simulink model "Decoder_3_8"  (R2018a)
settings: Solver=VariableStepAuto  StartTime=0.0  StopTime=10.0  RelTol=1e-3
settings Model: Creator=midog  LastModifiedBy=midog

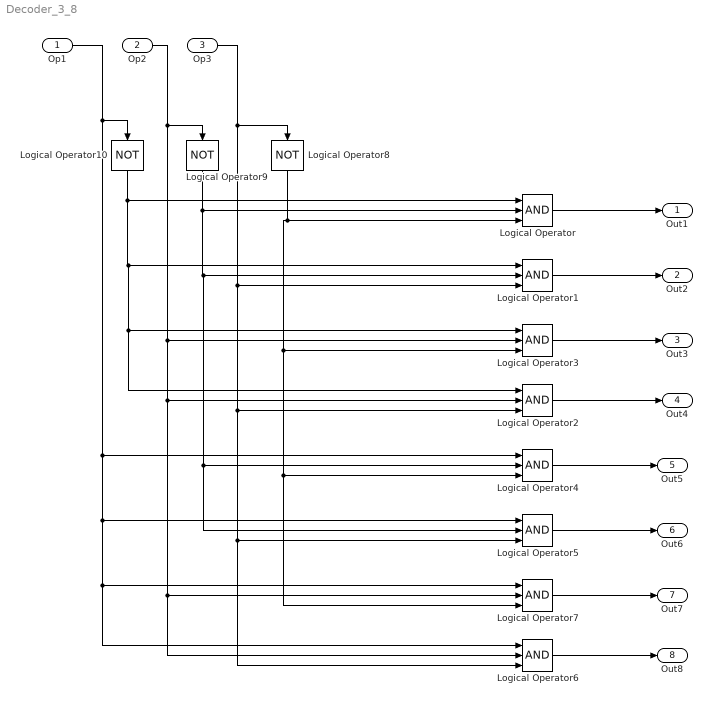
== system Decoder_3_8 ==
  Op1 : Inport  OutMin=0  OutMax=1
  Op2 : Inport  Port=2  OutMin=0  OutMax=1
  Op3 : Inport  Port=3  OutMin=0  OutMax=1
  Logical Operator{,1..7} (8 alike) : Logic  Inputs=3  IconShape=distinctive  AllPortsSameDT=off  OutDataTypeStr=boolean
  Logical Operator10 : Logic  Operator=NOT  Inputs=1  IconShape=distinctive  AllPortsSameDT=off  OutDataTypeStr=boolean
  Logical Operator8 : Logic  Operator=NOT  Inputs=1  IconShape=distinctive  AllPortsSameDT=off  OutDataTypeStr=boolean
  Logical Operator9 : Logic  Operator=NOT  Inputs=1  IconShape=distinctive  AllPortsSameDT=off  OutDataTypeStr=boolean
  Out1 : Outport
  Out2 : Outport  Port=2
  Out3 : Outport  Port=3
  Out4 : Outport  Port=4
  Out5 : Outport  Port=5
  Out6 : Outport  Port=6
  Out7 : Outport  Port=7
  Out8 : Outport  Port=8
  wires:
  Logical Operator10/1 -> Logical Operator2/1, Logical Operator3/1, Logical Operator1/1, Logical Operator/1
  Op3/1 -> Logical Operator8/1, Logical Operator1/3, Logical Operator2/3, Logical Operator6/3, Logical Operator5/3
  Logical Operator9/1 -> Logical Operator/2, Logical Operator1/2, Logical Operator5/2, Logical Operator4/2
  Op2/1 -> Logical Operator3/2, Logical Operator2/2, Logical Operator6/2, Logical Operator7/2, Logical Operator9/1
  Logical Operator8/1 -> Logical Operator3/3, Logical Operator7/3, Logical Operator4/3, Logical Operator/3
  Op1/1 -> Logical Operator4/1, Logical Operator5/1, Logical Operator7/1, Logical Operator6/1, Logical Operator10/1
  Logical Operator/1 -> Out1/1
  Logical Operator1/1 -> Out2/1
  Logical Operator3/1 -> Out3/1
  Logical Operator2/1 -> Out4/1
  Logical Operator4/1 -> Out5/1
  Logical Operator5/1 -> Out6/1
  Logical Operator7/1 -> Out7/1
  Logical Operator6/1 -> Out8/1
